simulink model "clik_inverse"  (R2022b)
settings: Solver=ode1  StartTime=0.0  StopTime=4  FixedStep=0.001  RelTol=1e-3
undefined symbols (not defined in the file or in its folder): DiscIntNeverNeededParam, q0, Tc
settings Model: Creator=Xp  LastModifiedBy=CHINMAY PRASHANTH
settings SolverCC: AlgebraicLoopSolver=TrustRegion
settings DataIOCC: LimitDataPoints=on  SaveFormat=Array  SignalLoggingSaveFormat=ModelDataLogs  ReturnWorkspaceOutputs=off
settings OptimizationCC: ExpressionDepthLimit=2147483647  InitFltsAndDblsToZero=on  LifeSpan=inf
settings DebuggingCC: SaveWithParameterizedLinksMsg=none  UnderspecifiedInitializationDetection=Classic  MergeDetectMultiDrivingBlocksExec=none  SolverPrmCheckMsg=warning  MultiTaskDSMMsg=warning  MultiTaskCondExecSysMsg=none  FcnCallInpInsideContextMsg=warning  UnconnectedInputMsg=warning  UnconnectedOutputMsg=warning  UnconnectedLineMsg=warning  StateNameClashWarn=warning  SFUnexpectedBacktrackingDiag=warning  SFNoUnconditionalDefaultTransitionDiag=warning  SFExecutionAtInitializationDiag=none  SFMachineParentedDataDiag=warning  ArithmeticOperatorsInVariantConditions=warning
settings HardwareCC: ProdBitPerPointer=32  ProdBitPerSizeT=32  ProdBitPerPtrDiffT=32  ProdLargestAtomicFloat=None  ProdIntDivRoundTo=Undefined  ProdEndianess=Unspecified  ProdWordSize=32  ProdHWDeviceType=32-bit Generic
settings ModelReferenceCC: EnableRefExpFcnMdlSchedulingChecks=on  PropagateSignalLabelsOutOfModel=off
settings SFSimCC: CustomCodeUndefinedFunction=UseInterfaceOnly
settings RTWCC: DLArmComputeVersion=19.05
settings CodeAppCC: StateflowObjectComments=on
settings GRTTargetCC: TargetLangStandard=C89/C90 (ANSI)  CombineOutputUpdateFcns=off  GRTInterface=on
settings ConfigComp: CovMetricSettings=dw  CovSaveCumulativeToWorkspaceVar=on  CovSaveSingleToWorkspaceVar=on

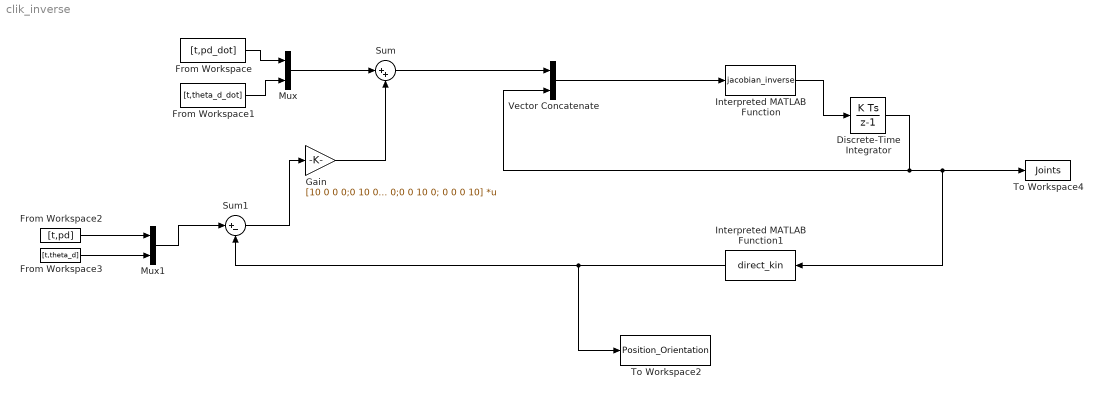
== system clik_inverse ==
  Discrete-Time Integrator : DiscreteIntegrator  InitialCondition=q0  SampleTime=Tc  ICPrevOutput=DiscIntNeverNeededParam  ICPrevScaledInput=DiscIntNeverNeededParam
  From Workspace : FromWorkspace  VariableName=[t,pd_dot]  SampleTime=Tc
  From Workspace1 : FromWorkspace  VariableName=[t,theta_d_dot]
  From Workspace2 : FromWorkspace  VariableName=[t,pd]
  From Workspace3 : FromWorkspace  VariableName=[t,theta_d]
  Gain : Gain  Gain=[10 0 0 0;0 10 0 0;0 0 10 0; 0 0 0 10]  Multiplication=Matrix(K*u)
  Interpreted MATLAB Function : MATLABFcn  MATLABFcn=jacobian_inverse  OutputDimensions=4
  Interpreted MATLAB Function1 : MATLABFcn  MATLABFcn=direct_kin  OutputDimensions=4
  Mux : Mux  Inputs=2
  Mux1 : Mux  Inputs=2
  Sum : Sum  Inputs=|++
  Sum1 : Sum  Inputs=|+-
  To Workspace2 : ToWorkspace  VariableName=Position_Orientation  SampleTime=-1
  To Workspace4 : ToWorkspace  VariableName=Joints  SampleTime=-1
  Vector Concatenate : Concatenate
  wires:
  Vector Concatenate/1 -> Interpreted MATLAB Function/1
  From Workspace/1 -> Mux/1
  From Workspace1/1 -> Mux/2
  Mux/1 -> Sum/1
  Gain/1 -> Sum/2
  Sum/1 -> Vector Concatenate/1
  Discrete-Time Integrator/1 -> Vector Concatenate/2, Interpreted MATLAB Function1/1, To Workspace4/1
  Sum1/1 -> Gain/1
  Mux1/1 -> Sum1/1
  From Workspace2/1 -> Mux1/1
  From Workspace3/1 -> Mux1/2
  Interpreted MATLAB Function1/1 -> To Workspace2/1, Sum1/2
  Interpreted MATLAB Function/1 -> Discrete-Time Integrator/1
